simulink library "TEsim_utils"  (R2013b)
settings: Solver=ode45  StartTime=0.0  StopTime=10.0  RelTol=1e-3
undefined symbols (not defined in the file): Dprocplc, IDVspec, r1_0, r4_0, tesim_ic, Ts_base, Ts_scan
libraries: TElib x17, instrumentlib x2, simulink_extras x1
settings Model: Creator=rnc4  LastModifiedBy=rnc4

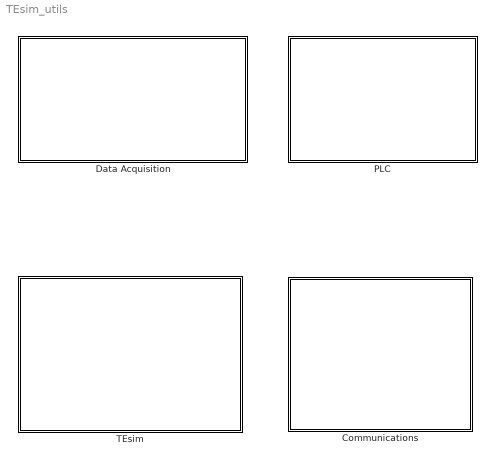
== system TEsim_utils ==
  Communications : Subsystem
      mask Display: image('comms.gif')
  Data Acquisition : Subsystem
      mask Display: image('das.jpg')
  PLC : Subsystem
      mask Display: image('CX1020.jpg')
  TEsim : Subsystem
      mask Display: image('te_sim.jpg')

== system TEsim_utils/Communications ==
  Receive Signal UDP : Subsystem  mask{Host=localhost, Port=9901, LocalPort=-1, SampleTime=0.01}
      mask prompts: LocalPort "Local port:"; SampleTime "Block sample time:"
      mask TypeOptions Host: UDP Receive/Host
      mask TypeOptions Port: UDP Receive/Port
      mask TypeOptions LocalPort: UDP Receive/LocalPort
      mask TypeOptions SampleTime: UDP Receive/SampleTime
      mask Display: text(0.25,0.5,'Recv UDP')
  Transmit Signal UDP : Subsystem  mask{Ts=0, Host=localhost, Port=9901, LocalPort=-1, EnableBlockingMode=on}
      mask prompts: Ts "Sample time:"; Port "Remote Port:"; LocalPort "Local Port:"; EnableBlockingMode "Enable blocking mode"
      mask TypeOptions Host: UDP Send/Host
      mask TypeOptions Port: UDP Send/Port
      mask TypeOptions LocalPort: UDP Send/LocalPort
      mask TypeOptions EnableBlockingMode: UDP Send/EnableBlockingMode
      mask Display: text(0.25,0.5,'Send UDP')

== system TEsim_utils/Data Acquisition ==
  DAQ : Subsystem  mask(DAQ without ADC){frame_dur_sec=1, timeslot_offset_ms=10}
      mask prompts: frame_dur_sec "Frame duration (sec):"; timeslot_offset_ms "Timeslot offset (ms):"
      mask help:
      | This block emulates data acquistion and transmission of sensor values over a timeslotted (TDMA) medium such as WirelessHART or ISA100.11a.
      |
      | The frame duration is specified in seconds as "Frame Duration".  This parameter may be considered how often the sensor value is latched and transmitted.  Sensor readings are taken at the precise moment that the transmission is made.
      |
      | The timeslot is specified in milliseconds and must be smaller than that frame duration.
      mask Display:
      | port_label('input',1,'x(t)')
      | port_label('output',1,'x[k]')
      | 
      | text(.5,.5,'DAQ: x(t) \rightarrow x[k]','hor','center','texmode','on')
  DAQ with 0-5 V 12-bit quatizer : Subsystem  mask(DAQ with Idealized ADC){frame_dur_sec=1, timeslot_offset_ms=10, NumberOfConverterBits=12, Vmin=0, Vmax=5, Gain=1}
      mask prompts: frame_dur_sec "Frame duration (sec):"; timeslot_offset_ms "Timeslot offset (ms):"; NumberOfConverterBits "SimulinkBlocks:simulink_extras:NumberOfConverterBits_MP"; Vmin "SimulinkBlocks:simulink_extras:MinInputVoltageAtLowOutput_MP"; Vmax "SimulinkBlocks:simulink_extras:MaxInputVoltageAt2nOutputunreachable_MP"; Gain "Input scaling gain:"
      mask help:
      | This block emulates data acquistion and transmission of sensor values over a timeslotted (TDMA) medium such as WirelessHART or ISA100.11a.
      |
      | The frame duration is specified in seconds as "Frame Duration".  This parameter may be considered how often the sensor value is latched and transmitted.  Sensor readings are taken at the precise moment that the transmission is made.
      |
      | The timeslot is specified in milliseconds and must be smaller than that frame duration.
      |
      | The ADC parameters are as follows:
      | * Number of bits used by the ADC. Default is 12 bits.
      | * Voltage low and high values.  Note that although voltage is specified, it could as well be current.
      | * Negative values are not allowed.
      mask TypeOptions NumberOfConverterBits: Idealized ADC quantizer/NumberOfConverterBits
      mask TypeOptions Vmin: Idealized ADC quantizer/Vmin
      mask TypeOptions Vmax: Idealized ADC quantizer/Vmax
      mask TypeOptions Gain: Gain/Gain
      mask Display:
      | port_label('input',1,'x(t)')
      | port_label('output',1,'x[k]')
      | 
      | text(.5,.5,'DAQ: x(t) \rightarrow x[k]','hor','center','texmode','on')

== system TEsim_utils/PLC ==
  TE Controller PLC Input : Subsystem  mask{SampleTime=Ts_scan}
      mask prompts: SampleTime "Sample time (-1 for inherited):"
      mask TypeOptions SampleTime:
      | Zero-Order
      | Hold/SampleTime
  TEController PLC Output : Subsystem  mask{DelayTime=Dprocplc, InitialOutput=1}
      mask prompts: DelayTime "PLC Processing Delay:"; InitialOutput "Initial output:"
      mask TypeOptions DelayTime:
      | Transport
      | Delay/DelayTime
      mask TypeOptions InitialOutput:
      | Transport
      | Delay/InitialOutput

== system TEsim_utils/TEsim ==
  Controller : Subsystem
  TE Plant : Subsystem  mask{tesim_ic=tesim_ic}
      mask prompts: tesim_ic "Plant ic:"
      mask TypeOptions tesim_ic: TE Plant Model/tesim_ic

== system TEsim_utils/Communications/Receive Signal UDP ==
  Terminator : Terminator
  UDP Receive : instrumentlib/UDP Receive  Host=localhost  Port=Port  LocalPort=LocalPort  DataSize=[1 1]  EnableBlockingMode=off  Timeout=10  SampleTime=SampleTime  DataType=double  ByteOrder=BigEndian
  x : Outport
  wires:
  UDP Receive/2 -> Terminator/1
  UDP Receive/1 -> x/1

== system TEsim_utils/Communications/Transmit Signal UDP ==
  x : Inport
  Rate Transition : RateTransition  OutPortSampleTime=Ts
  UDP Send : instrumentlib/UDP Send  Host=localhost  Port=Port  LocalPort=LocalPort  EnableBlockingMode=on  ByteOrder=BigEndian
  wires:
  Rate Transition/1 -> UDP Send/1
  x/1 -> Rate Transition/1

== system TEsim_utils/Data Acquisition/DAQ ==
  note: Input Value
  note: Output Value
  Analog In : Inport
  Rate Transition : RateTransition  Deterministic=off  OutPortSampleTime=[frame_dur_sec timeslot_offset_ms/1000]
      settings: AttributesFormatString=Ts_o = %<OutPortSampleTime>
  Digital Out : Outport
  wires:
  Rate Transition/1 -> Digital Out/1
  Analog In/1 -> Rate Transition/1

== system TEsim_utils/Data Acquisition/DAQ with 0-5 V 12-bit quatizer ==
  note: Output Value
  note: Input Value
  Analog In : Inport
  Gain : Gain  Gain=Gain
  Idealized ADC quantizer : simulink_extras/Additional Discrete/Idealized ADC quantizer  NumberOfConverterBits=NumberOfConverterBits  Vmin=Vmin  Vmax=Vmax  OutputDataType=int16  OutputNegativeValues=off
  Rate Transition : RateTransition  Deterministic=off  OutPortSampleTime=[frame_dur_sec timeslot_offset_ms/1000]
      settings: AttributesFormatString=Ts_o = %<OutPortSampleTime>
  Digital Out : Outport
  wires:
  Analog In/1 -> Gain/1
  Rate Transition/1 -> Digital Out/1
  Idealized ADC quantizer/1 -> Rate Transition/1
  Gain/1 -> Idealized ADC quantizer/1

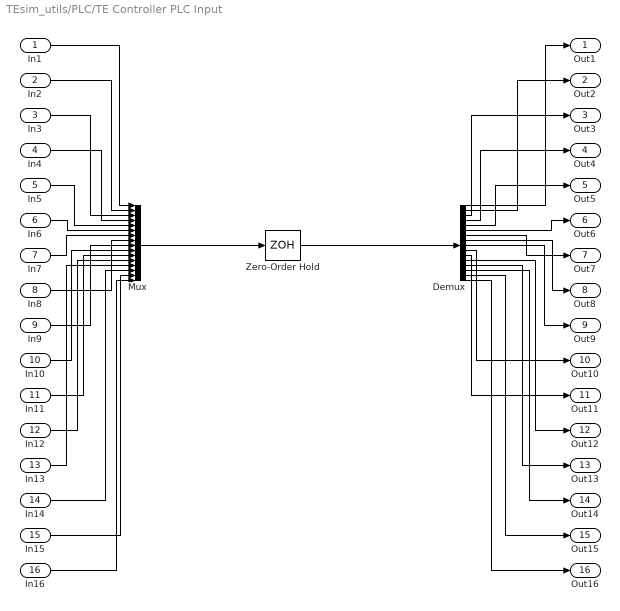
== system TEsim_utils/PLC/TE Controller PLC Input ==
  In1 : Inport
  In2 : Inport  Port=2
  In3 : Inport  Port=3
  In4 : Inport  Port=4
  In5 : Inport  Port=5
  In6 : Inport  Port=6
  In7 : Inport  Port=7
  In8 : Inport  Port=8
  In9 : Inport  Port=9
  In10 : Inport  Port=10
  In11 : Inport  Port=11
  In12 : Inport  Port=12
  In13 : Inport  Port=13
  In14 : Inport  Port=14
  In15 : Inport  Port=15
  In16 : Inport  Port=16
  Demux : Demux  Outputs=16
  Mux : Mux  Inputs=16
  Zero-Order Hold : ZeroOrderHold  SampleTime=SampleTime
  Out1 : Outport
  Out2 : Outport  Port=2
  Out3 : Outport  Port=3
  Out4 : Outport  Port=4
  Out5 : Outport  Port=5
  Out6 : Outport  Port=6
  Out7 : Outport  Port=7
  Out8 : Outport  Port=8
  Out9 : Outport  Port=9
  Out10 : Outport  Port=10
  Out11 : Outport  Port=11
  Out12 : Outport  Port=12
  Out13 : Outport  Port=13
  Out14 : Outport  Port=14
  Out15 : Outport  Port=15
  Out16 : Outport  Port=16
  wires:
  In16/1 -> Mux/16
  In1/1 -> Mux/1
  Demux/4 -> Out4/1
  In3/1 -> Mux/3
  In12/1 -> Mux/12
  In9/1 -> Mux/9
  Demux/5 -> Out5/1
  In5/1 -> Mux/5
  In14/1 -> Mux/14
  Demux/14 -> Out14/1
  In15/1 -> Mux/15
  In10/1 -> Mux/10
  In4/1 -> Mux/4
  In13/1 -> Mux/13
  In6/1 -> Mux/6
  Demux/16 -> Out16/1
  Demux/9 -> Out9/1
  In2/1 -> Mux/2
  In7/1 -> Mux/7
  In8/1 -> Mux/8
  In11/1 -> Mux/11
  Demux/10 -> Out10/1
  Demux/11 -> Out11/1
  Demux/13 -> Out13/1
  Demux/12 -> Out12/1
  Mux/1 -> Zero-Order Hold/1
  Demux/1 -> Out1/1
  Demux/2 -> Out2/1
  Demux/7 -> Out7/1
  Demux/8 -> Out8/1
  Demux/3 -> Out3/1
  Demux/6 -> Out6/1
  Demux/15 -> Out15/1
  Zero-Order Hold/1 -> Demux/1

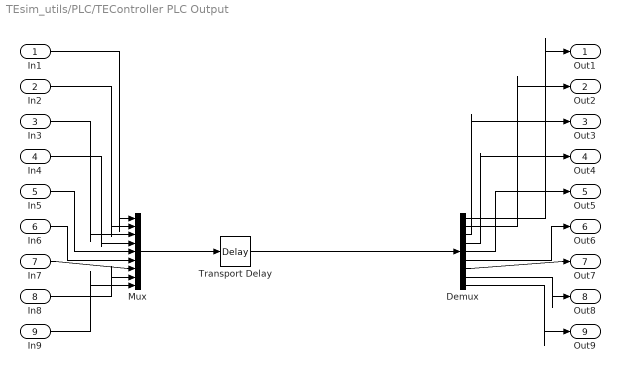
== system TEsim_utils/PLC/TEController PLC Output ==
  In1 : Inport
  In2 : Inport  Port=2
  In3 : Inport  Port=3
  In4 : Inport  Port=4
  In5 : Inport  Port=5
  In6 : Inport  Port=6
  In7 : Inport  Port=7
  In8 : Inport  Port=8
  In9 : Inport  Port=9
  Demux : Demux  Outputs=9
  Mux : Mux  Inputs=9
  Transport Delay : TransportDelay  DelayTime=DelayTime  InitialOutput=InitialOutput
  Out1 : Outport
  Out2 : Outport  Port=2
  Out3 : Outport  Port=3
  Out4 : Outport  Port=4
  Out5 : Outport  Port=5
  Out6 : Outport  Port=6
  Out7 : Outport  Port=7
  Out8 : Outport  Port=8
  Out9 : Outport  Port=9
  wires:
  Transport Delay/1 -> Demux/1
  Demux/6 -> Out6/1
  Demux/3 -> Out3/1
  Demux/8 -> Out8/1
  Demux/7 -> Out7/1
  Demux/2 -> Out2/1
  Demux/1 -> Out1/1
  Mux/1 -> Transport Delay/1
  In8/1 -> Mux/8
  In7/1 -> Mux/7
  In2/1 -> Mux/2
  Demux/9 -> Out9/1
  In6/1 -> Mux/6
  In4/1 -> Mux/4
  In5/1 -> Mux/5
  Demux/5 -> Out5/1
  In9/1 -> Mux/9
  In3/1 -> Mux/3
  Demux/4 -> Out4/1
  In1/1 -> Mux/1

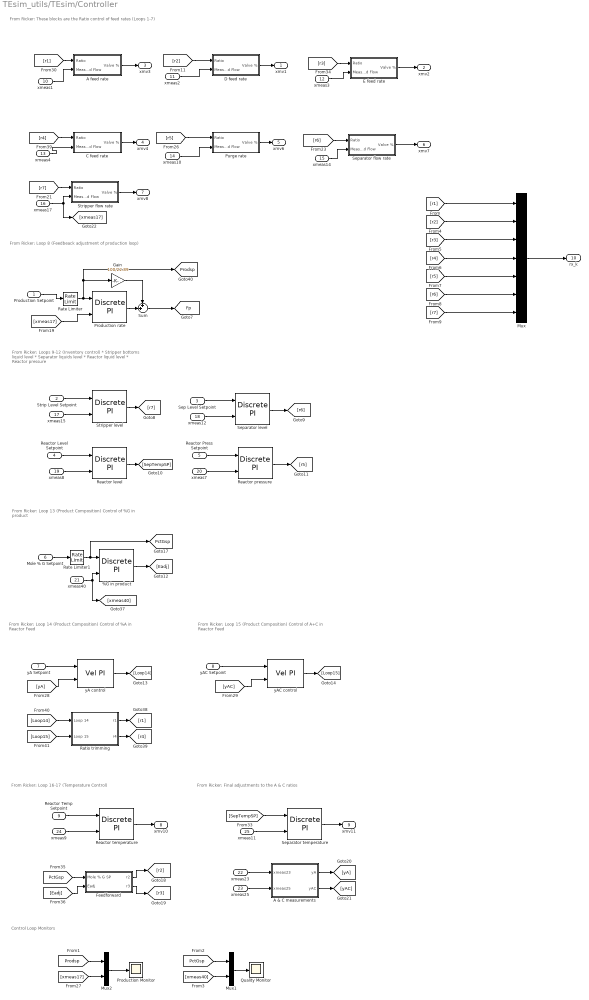
== system TEsim_utils/TEsim/Controller ==
  note: From Ricker: These blocks are the Ratio control of feed rates (Loops 1-7)
  note: From Ricker: Loop 8 (Feedbeack adjustment of production loop)
  note: From Ricker: Loops 9-12 (Inventory control)
      | * Stripper bottoms liquid level
      | * Separator liquids level
      | * Reactor liquid level
      | * Reactor pressure
  note: From Ricker: Loop 13 (Product Composition)
      | Control of %G in product
  note: From Ricker: Loop 16-17 (Temperature Control)
  note: From Ricker: Loop 14 (Product Composition)
      | Control of %A in Reactor Feed
  note: From Ricker: Loop 15 (Product Composition)
      | Control of A+C in Reactor Feed
  note: From Ricker: Final adjustments to the A & C ratios
  note: Control Loop Monitors
  Production Setpoint : Inport
  Strip Level Setpoint : Inport  Port=2
  Sep Level Setpoint : Inport  Port=3
  Reactor Level Setpoint : Inport  Port=4
  Reactor Press Setpoint : Inport  Port=5
  Mole % G Setpoint : Inport  Port=6
  yA Setpoint : Inport  Port=7
  yAC Setpoint : Inport  Port=8
  Reactor Temp Setpoint : Inport  Port=9
  xmeas1 : Inport  Port=10
  xmeas2 : Inport  Port=11
  xmeas3 : Inport  Port=12
  xmeas4 : Inport  Port=13
  xmeas10 : Inport  Port=14
  xmeas14 : Inport  Port=15
  xmeas17 : Inport  Port=16
  xmeas15 : Inport  Port=17
  xmeas12 : Inport  Port=18
  xmeas8 : Inport  Port=19
  xmeas7 : Inport  Port=20
  xmeas40 : Inport  Port=21
  xmeas23 : Inport  Port=22
  xmeas25 : Inport  Port=23
  xmeas9 : Inport  Port=24
  xmeas11 : Inport  Port=25
  %G in product : TElib/Discrete PI  Kc=-0.4  Ti=100/60  Ts=Ts_base  x0=Eadj_0  Hi=inf  Lo=-inf
  A & C measurements : Subsystem
  A feed rate : Subsystem
  C feed rate : Subsystem
  D feed rate : Subsystem
  E feed rate : Subsystem
  Feedforward : Subsystem
  Gain : Gain  Gain=100/22.89  SaturateOnIntegerOverflow=on  OutDataTypeStr=Inherit: Same as input  ParamDataTypeStr=Inherit: Same as input
  Mux : Mux  Inputs=7
  Mux1 : Mux  Inputs=2
  Mux2 : Mux  Inputs=2
  Production Monitor : Scope
      settings: YMin=20  YMax=28  SaveName=Production  SampleInput=on  SampleTime=Ts_save
  Production rate : TElib/Discrete PI  Kc=3.2  Ti=120/60  Ts=Ts_base  x0=0  Hi=30  Lo=-30
  Purge rate : Subsystem
  Quality Monitor : Scope
      settings: YMin=40  YMax=60  SaveName=Quality  SampleInput=on  SampleTime=Ts_save
  Rate Limiter : RateLimiter  RisingSlewLimit=0.3*22.95/24  FallingSlewLimit=-0.3*22.95/24
  Rate Limiter1 : RateLimiter  RisingSlewLimit=50/24  FallingSlewLimit=-50/24
  Ratio trimming : Subsystem
  Reactor level : TElib/Discrete PI  Kc=0.8  Ti=60/60  Ts=Ts_base  x0=SP17_0  Hi=120  Lo=0
  Reactor pressure : TElib/Discrete PI  Kc=-1e-4  Ti=20/60  Ts=Ts_base  x0=r5_0  Hi=100  Lo=0
  Reactor temperature : TElib/Discrete PI  Kc=-8  Ti=7.5/60  Ts=Ts_base  x0=xmv10_0  Hi=100  Lo=0
  Separator flow rate : Subsystem
  Separator level : TElib/Discrete PI  Kc=-1e-3  Ti=200/60  Ts=Ts_base  x0=r6_0  Hi=100  Lo=0
  Separator temperature : TElib/Discrete PI  Kc=-4  Ti=15/60  Ts=Ts_base  x0=xmv11_0  Hi=100  Lo=0
  Stripper flow rate : Subsystem
  Stripper level : TElib/Discrete PI  Kc=-2e-4  Ti=200/60  Ts=Ts_base  x0=r7_0  Hi=100  Lo=0
  Sum : Sum  Inputs=++|  SaturateOnIntegerOverflow=on
  yA control : TElib/Discrete PI/Vel PI  Kc=2e-4  Ti=1  Ts=0.1
  yAC control : TElib/Discrete PI/Vel PI  Kc=3e-4  Ti=2  Ts=0.1
  xmv1 : Outport
  xmv2 : Outport  Port=2
  xmv3 : Outport  Port=3
  xmv4 : Outport  Port=4
  xmv6 : Outport  Port=5
  xmv7 : Outport  Port=6
  xmv8 : Outport  Port=7
  xmv10 : Outport  Port=8
  xmv11 : Outport  Port=9
  rx_k : Outport  Port=10
  tag scope: Fp=global, PctGsp=global, Prodsp=global
  wires:
  Ratio trimming/1(r1) -> [r1]
  yA control/1 -> [Loop14]
  Ratio trimming/2(r4) -> [r4]
  [Loop15] -> Ratio trimming/2(Loop 15)
  Strip Level Setpoint/1 -> Stripper level/1
  [yAC] -> yAC control/2
  [Loop14] -> Ratio trimming/1(Loop 14)
  Production rate/1 -> Sum/2
  [Eadj] -> Feedforward/2(Eadj)
  Reactor level/1 -> [SepTempSP]
  [r6] -> Separator flow rate/1(Ratio)
  xmeas10/1 -> Purge rate/2(Measured Flow)
  Gain/1 -> Sum/1
  [r7] -> Stripper flow rate/1(Ratio)
  xmeas14/1 -> Separator flow rate/2(Measured Flow)
  Reactor Press Setpoint/1 -> Reactor pressure/1
  yAC Setpoint/1 -> yAC control/1
  [r2] -> D feed rate/1(Ratio)
  Reactor Level Setpoint/1 -> Reactor level/1
  [r1] -> A feed rate/1(Ratio)
  xmeas17/1 -> [xmeas17], Stripper flow rate/2(Measured Flow)
  [PctGsp] -> Feedforward/1(Mole % G SP)
  Production Setpoint/1 -> Rate Limiter/1
  [r4] -> C feed rate/1(Ratio)
  [yA] -> yA control/2
  [r3] -> E feed rate/1(Ratio)
  Reactor Temp Setpoint/1 -> Reactor temperature/1
  [r5] -> Purge rate/1(Ratio)
  Mole % G Setpoint/1 -> Rate Limiter1/1
  %G in product/1 -> [Eadj]
  [SepTempSP] -> Separator temperature/1
  Reactor pressure/1 -> [r5]
  A & C measurements/1(yA) -> [yA]
  xmeas1/1 -> A feed rate/2(Measured Flow)
  Feedforward/1(r2) -> [r2]
  Rate Limiter/1 -> Production rate/1, [Prodsp], Gain/1
  A & C measurements/2(yAC) -> [yAC]
  Feedforward/2(r3) -> [r3]
  Stripper level/1 -> [r7]
  Separator level/1 -> [r6]
  Rate Limiter1/1 -> %G in product/1, [PctGsp]
  Sep Level Setpoint/1 -> Separator level/1
  Sum/1 -> [Fp]
  yAC control/1 -> [Loop15]
  yA Setpoint/1 -> yA control/1
  xmeas2/1 -> D feed rate/2(Measured Flow)
  xmeas3/1 -> E feed rate/2(Measured Flow)
  xmeas4/1 -> C feed rate/2(Measured Flow)
  [xmeas17] -> Production rate/2
  xmeas15/1 -> Stripper level/2
  xmeas12/1 -> Separator level/2
  xmeas8/1 -> Reactor level/2
  xmeas7/1 -> Reactor pressure/2
  xmeas40/1 -> [xmeas40], %G in product/2
  xmeas23/1 -> A & C measurements/1(xmeas23)
  xmeas25/1 -> A & C measurements/2(xmeas25)
  xmeas9/1 -> Reactor temperature/2
  xmeas11/1 -> Separator temperature/2
  A feed rate/1(Valve %) -> xmv3/1
  D feed rate/1(Valve %) -> xmv1/1
  E feed rate/1(Valve %) -> xmv2/1
  C feed rate/1(Valve %) -> xmv4/1
  Purge rate/1(Valve %) -> xmv6/1
  Separator flow rate/1(Valve %) -> xmv7/1
  Stripper flow rate/1(Valve %) -> xmv8/1
  Reactor temperature/1 -> xmv10/1
  Separator temperature/1 -> xmv11/1
  [Prodsp] -> Mux2/1
  [xmeas17] -> Mux2/2
  Mux2/1 -> Production Monitor/1
  [PctGsp] -> Mux1/1
  [xmeas40] -> Mux1/2
  Mux1/1 -> Quality Monitor/1
  [r7] -> Mux/7
  [r2] -> Mux/2
  [r3] -> Mux/3
  [r4] -> Mux/4
  [r5] -> Mux/5
  [r6] -> Mux/6
  [r1] -> Mux/1
  Mux/1 -> rx_k/1

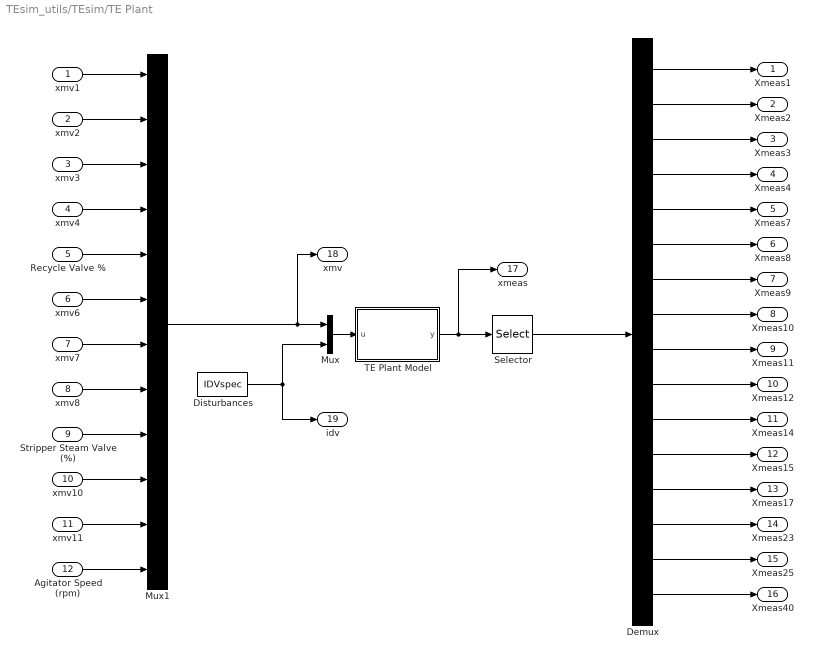
== system TEsim_utils/TEsim/TE Plant ==
  xmv1 : Inport
  xmv2 : Inport  Port=2
  xmv3 : Inport  Port=3
  xmv4 : Inport  Port=4
  Recycle Valve % : Inport  Port=5
  xmv6 : Inport  Port=6
  xmv7 : Inport  Port=7
  xmv8 : Inport  Port=8
  Stripper Steam Valve (%) : Inport  Port=9
  xmv10 : Inport  Port=10
  xmv11 : Inport  Port=11
  Agitator Speed (rpm) : Inport  Port=12
  Demux : Demux  Outputs=16
  Disturbances : Constant  Value=IDVspec  SampleTime=Ts_base
  Mux : Mux  Inputs=2
  Mux1 : Mux  Inputs=12
  Selector : Selector  InputPortWidth=41  IndexOptions=Index vector (dialog)  Indices=[1:4, 7:12, 14, 15, 17, 23, 25, 40]  OutputSizes=1
  TE Plant Model : Subsystem  mask{tesim_ic=tesim_ic}
      mask prompts: tesim_ic "Plant ic:"
  Xmeas1 : Outport
  Xmeas2 : Outport  Port=2
  Xmeas3 : Outport  Port=3
  Xmeas4 : Outport  Port=4
  Xmeas7 : Outport  Port=5
  Xmeas8 : Outport  Port=6
  Xmeas9 : Outport  Port=7
  Xmeas10 : Outport  Port=8
  Xmeas11 : Outport  Port=9
  Xmeas12 : Outport  Port=10
  Xmeas14 : Outport  Port=11
  Xmeas15 : Outport  Port=12
  Xmeas17 : Outport  Port=13
  Xmeas23 : Outport  Port=14
  Xmeas25 : Outport  Port=15
  Xmeas40 : Outport  Port=16
  xmeas : Outport  Port=17
  xmv : Outport  Port=18
  idv : Outport  Port=19
  wires:
  Demux/14 -> Xmeas23/1
  Demux/15 -> Xmeas25/1
  Demux/10 -> Xmeas12/1
  Demux/9 -> Xmeas11/1
  Demux/8 -> Xmeas10/1
  Demux/16 -> Xmeas40/1
  Demux/11 -> Xmeas14/1
  Demux/13 -> Xmeas17/1
  Demux/12 -> Xmeas15/1
  Demux/7 -> Xmeas9/1
  Demux/2 -> Xmeas2/1
  Demux/4 -> Xmeas4/1
  Demux/3 -> Xmeas3/1
  Demux/5 -> Xmeas7/1
  Demux/6 -> Xmeas8/1
  Demux/1 -> Xmeas1/1
  Selector/1 -> Demux/1
  xmv11/1 -> Mux1/11
  xmv6/1 -> Mux1/6
  xmv10/1 -> Mux1/10
  Mux1/1 -> xmv/1, Mux/1
  xmv4/1 -> Mux1/4
  Disturbances/1 -> idv/1, Mux/2
  Recycle Valve %/1 -> Mux1/5
  Stripper Steam Valve (%)/1 -> Mux1/9
  Agitator Speed (rpm)/1 -> Mux1/12
  xmv8/1 -> Mux1/8
  xmv1/1 -> Mux1/1
  xmv3/1 -> Mux1/3
  xmv7/1 -> Mux1/7
  xmv2/1 -> Mux1/2
  TE Plant Model/1(y) -> Selector/1, xmeas/1
  Mux/1 -> TE Plant Model/1(u)

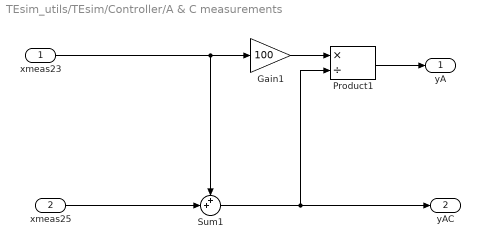
== system TEsim_utils/TEsim/Controller/A & C measurements ==
  xmeas23 : Inport
  xmeas25 : Inport  Port=2
  Gain1 : Gain  Gain=100  SaturateOnIntegerOverflow=on  OutDataTypeStr=Inherit: Same as input  ParamDataTypeStr=Inherit: Same as input
  Product1 : Product  Inputs=*/  SaturateOnIntegerOverflow=on  OutDataTypeStr=Inherit: Same as first input
  Sum1 : Sum  Inputs=++|  SaturateOnIntegerOverflow=on
  yA : Outport
  yAC : Outport  Port=2
  wires:
  Sum1/1 -> yAC/1, Product1/2
  xmeas23/1 -> Sum1/1, Gain1/1
  xmeas25/1 -> Sum1/2
  Gain1/1 -> Product1/1
  Product1/1 -> yA/1

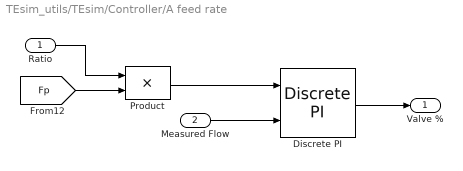
== system TEsim_utils/TEsim/Controller/A feed rate ==
  Ratio : Inport
  Measured Flow : Inport  Port=2
  Discrete PI : TElib/Discrete PI  Kc=0.01  Ti=0.001/60  Ts=Ts_base  x0=xmv3_0  Hi=100  Lo=0
  Product : Product  SaturateOnIntegerOverflow=on  OutDataTypeStr=Inherit: Same as first input
  Valve % : Outport
  wires:
  Discrete PI/1 -> Valve %/1
  Ratio/1 -> Product/1
  [Fp] -> Product/2
  Measured Flow/1 -> Discrete PI/2
  Product/1 -> Discrete PI/1

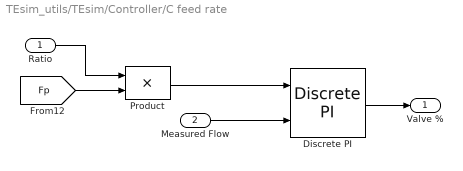
== system TEsim_utils/TEsim/Controller/C feed rate ==
  Ratio : Inport
  Measured Flow : Inport  Port=2
  Discrete PI : TElib/Discrete PI  Kc=0.003  Ti=0.001/60  Ts=Ts_base  x0=xmv4_0  Hi=100  Lo=0
  Product : Product  SaturateOnIntegerOverflow=on  OutDataTypeStr=Inherit: Same as first input
  Valve % : Outport
  wires:
  Product/1 -> Discrete PI/1
  Measured Flow/1 -> Discrete PI/2
  [Fp] -> Product/2
  Ratio/1 -> Product/1
  Discrete PI/1 -> Valve %/1

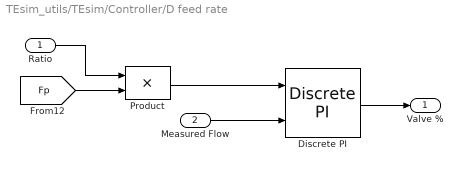
== system TEsim_utils/TEsim/Controller/D feed rate ==
  Ratio : Inport
  Measured Flow : Inport  Port=2
  Discrete PI : TElib/Discrete PI  Kc=1.6e-6  Ti=0.001/60  Ts=Ts_base  x0=xmv1_0  Hi=100  Lo=0
  Product : Product  SaturateOnIntegerOverflow=on  OutDataTypeStr=Inherit: Same as first input
  Valve % : Outport
  wires:
  Product/1 -> Discrete PI/1
  Measured Flow/1 -> Discrete PI/2
  [Fp] -> Product/2
  Ratio/1 -> Product/1
  Discrete PI/1 -> Valve %/1

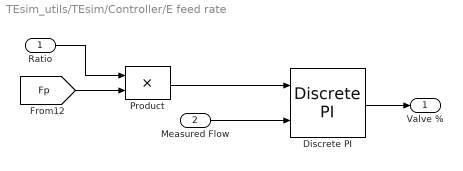
== system TEsim_utils/TEsim/Controller/E feed rate ==
  Ratio : Inport
  Measured Flow : Inport  Port=2
  Discrete PI : TElib/Discrete PI  Kc=1.8e-6  Ti=0.001/60  Ts=Ts_base  x0=xmv2_0  Hi=100  Lo=0
  Product : Product  SaturateOnIntegerOverflow=on  OutDataTypeStr=Inherit: Same as first input
  Valve % : Outport
  wires:
  Product/1 -> Discrete PI/1
  Measured Flow/1 -> Discrete PI/2
  [Fp] -> Product/2
  Ratio/1 -> Product/1
  Discrete PI/1 -> Valve %/1

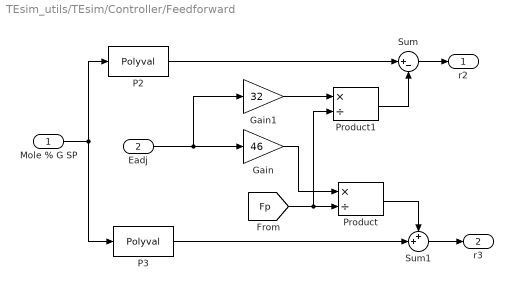
== system TEsim_utils/TEsim/Controller/Feedforward ==
  Mole % G SP : Inport
  Eadj : Inport  Port=2
  Gain : Gain  Gain=46  SaturateOnIntegerOverflow=on  OutDataTypeStr=Inherit: Same as input  ParamDataTypeStr=Inherit: Same as input
  Gain1 : Gain  Gain=32  SaturateOnIntegerOverflow=on  OutDataTypeStr=Inherit: Same as input  ParamDataTypeStr=Inherit: Same as input
  P2 : Polyval  Coefs="[1.5192e-003  5.9446e-001  2.7690e-001]"
  P3 : Polyval  Coefs="[-1.1377e-003 -8.0893e-001  9.1060e+001]"
  Product : Product  Inputs=*/  SaturateOnIntegerOverflow=on  OutDataTypeStr=Inherit: Same as first input
  Product1 : Product  Inputs=*/  SaturateOnIntegerOverflow=on  OutDataTypeStr=Inherit: Same as first input
  Sum : Sum  Inputs=|+-  SaturateOnIntegerOverflow=on
  Sum1 : Sum  Inputs=++|  SaturateOnIntegerOverflow=on
  r2 : Outport
  r3 : Outport  Port=2
  wires:
  Mole % G SP/1 -> P2/1, P3/1
  Sum/1 -> r2/1
  P2/1 -> Sum/1
  Sum1/1 -> r3/1
  P3/1 -> Sum1/2
  Product/1 -> Sum1/1
  [Fp] -> Product/2, Product1/2
  Gain/1 -> Product/1
  Eadj/1 -> Gain/1, Gain1/1
  Product1/1 -> Sum/2
  Gain1/1 -> Product1/1

== system TEsim_utils/TEsim/Controller/Purge rate ==
  Ratio : Inport
  Measured Flow : Inport  Port=2
  Discrete PI : TElib/Discrete PI  Kc=0.01  Ti=0.001/60  Ts=Ts_base  x0=xmv6_0  Hi=100  Lo=0
  Product : Product  SaturateOnIntegerOverflow=on  OutDataTypeStr=Inherit: Same as first input
  Valve % : Outport
  wires:
  Discrete PI/1 -> Valve %/1
  Ratio/1 -> Product/1
  [Fp] -> Product/2
  Measured Flow/1 -> Discrete PI/2
  Product/1 -> Discrete PI/1

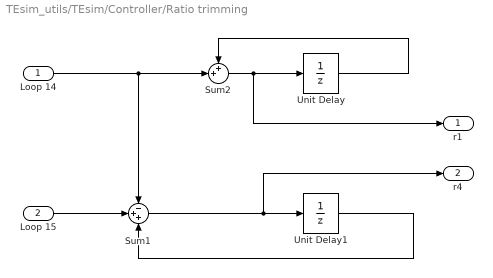
== system TEsim_utils/TEsim/Controller/Ratio trimming ==
  Loop 14 : Inport
  Loop 15 : Inport  Port=2
  Sum1 : Sum  Inputs=-++  SaturateOnIntegerOverflow=on
  Sum2 : Sum  Inputs=++|  SaturateOnIntegerOverflow=on
  Unit Delay : UnitDelay  InitialCondition=r1_0  SampleTime=0.1
  Unit Delay1 : UnitDelay  InitialCondition=r4_0  SampleTime=0.1
  r1 : Outport
  r4 : Outport  Port=2
  wires:
  Loop 15/1 -> Sum1/2
  Unit Delay/1 -> Sum2/1
  Unit Delay1/1 -> Sum1/3
  Sum2/1 -> Unit Delay/1, r1/1
  Loop 14/1 -> Sum2/2, Sum1/1
  Sum1/1 -> Unit Delay1/1, r4/1

== system TEsim_utils/TEsim/Controller/Separator flow rate ==
  Ratio : Inport
  Measured Flow : Inport  Port=2
  Discrete PI : TElib/Discrete PI  Kc=4e-4  Ti=0.001/60  Ts=Ts_base  x0=xmv7_0  Hi=100  Lo=0
  Product : Product  SaturateOnIntegerOverflow=on  OutDataTypeStr=Inherit: Same as first input
  Valve % : Outport
  wires:
  Product/1 -> Discrete PI/1
  Measured Flow/1 -> Discrete PI/2
  [Fp] -> Product/2
  Ratio/1 -> Product/1
  Discrete PI/1 -> Valve %/1

== system TEsim_utils/TEsim/Controller/Stripper flow rate ==
  Ratio : Inport
  Measured Flow : Inport  Port=2
  Discrete PI : TElib/Discrete PI  Kc=4e-4  Ti=0.001/60  Ts=Ts_base  x0=xmv8_0  Hi=100  Lo=0
  Product : Product  SaturateOnIntegerOverflow=on  OutDataTypeStr=Inherit: Same as first input
  Valve % : Outport
  wires:
  Discrete PI/1 -> Valve %/1
  Ratio/1 -> Product/1
  [Fp] -> Product/2
  Measured Flow/1 -> Discrete PI/2
  Product/1 -> Discrete PI/1

== system TEsim_utils/TEsim/TE Plant/TE Plant Model ==
  u : Inport
  TE Code : S-Function  FunctionName=temexd  Parameters=tesim_ic  EnableBusSupport=off
  y : Outport
  wires:
  u/1 -> TE Code/1
  TE Code/1 -> y/1
